simulink model "ex3c_simulink"  (R2025b)
settings: Solver=VariableStepAuto  StartTime=0.0  StopTime=10.0  RelTol=1e-3
undefined symbols (not defined in the file or in its folder): par3
settings Model: Creator=fred  LastModifiedBy=fred

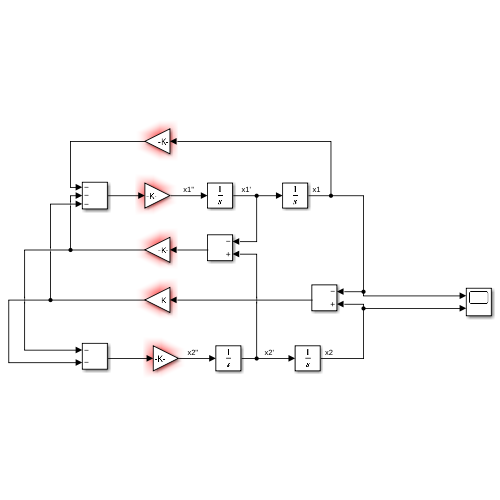
[thumbnail: Simulink's stored preview of the top-level diagram]
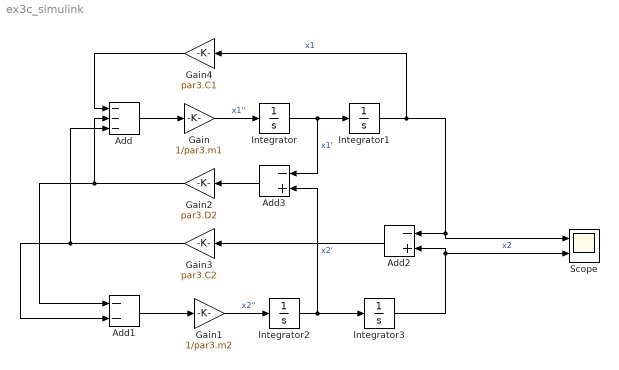
== system ex3c_simulink ==
  Add : Sum  Inputs=---
  Add1 : Sum  Inputs=--
  Add2 : Sum  Inputs=-+
  Add3 : Sum  Inputs=-+
  Gain : Gain  Gain=1/par3.m1
  Gain1 : Gain  Gain=1/par3.m2
  Gain2 : Gain  Gain=par3.D2
  Gain3 : Gain  Gain=par3.C2
  Gain4 : Gain  Gain=par3.C1
  Integrator{,1..3} (4 alike) : Integrator
  Scope : Scope  NumInputPorts=2
  wires:
  Integrator/1 -> Add3/1, Integrator1/1  "x1'"
  Gain/1 -> Integrator/1  "x1''"
  Integrator1/1 -> Gain4/1, Scope/1, Add2/1  "x1"
  Add/1 -> Gain/1
  Integrator2/1 -> Add3/2, Integrator3/1  "x2'"
  Integrator3/1 -> Scope/2, Add2/2  "x2"
  Gain1/1 -> Integrator2/1  "x2''"
  Add1/1 -> Gain1/1
  Gain4/1 -> Add/1
  Add2/1 -> Gain3/1
  Add3/1 -> Gain2/1
  Gain3/1 -> Add1/2, Add/3
  Gain2/1 -> Add1/1, Add/2
